simulink model "myLKS"  (R2013b)
settings: Solver=ode45  StartTime=0.0  StopTime=10.0  RelTol=1e-3
undefined symbols (not defined in the file or in its folder): A, B, GearRatio, K, L
settings Model: Creator=IVDL  LastModifiedBy=edward
settings DataIOCC: SignalLoggingSaveFormat=ModelDataLogs
settings DebuggingCC: UnderspecifiedInitializationDetection=Simplified  MultiTaskDSMMsg=warning  MultiTaskCondExecSysMsg=none  StrictBusMsg=None
settings RTWCC: IncludeERTFirstTime=on
settings GRTTargetCC: CodeReplacementLibrary=None  CPPClassGenCompliant=on

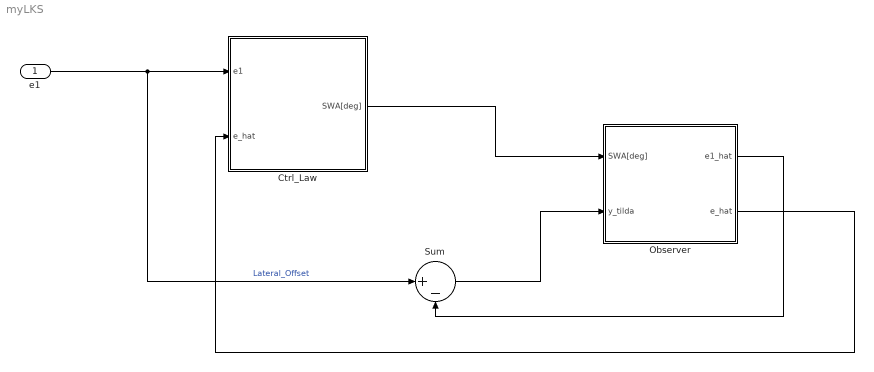
== system myLKS ==
  e1 : Inport
  Ctrl_Law : Subsystem
  Observer : Subsystem
  Sum : Sum  Inputs=|+-
  wires:
  Sum/1 -> Observer/2(y_tilda)
  e1/1 -> Sum/1, Ctrl_Law/1(e1)  "Lateral_Offset"
  Observer/2(e_hat) -> Ctrl_Law/2(e_hat)
  Ctrl_Law/1(SWA[deg]) -> Observer/1(SWA[deg])
  Observer/1(e1_hat) -> Sum/2

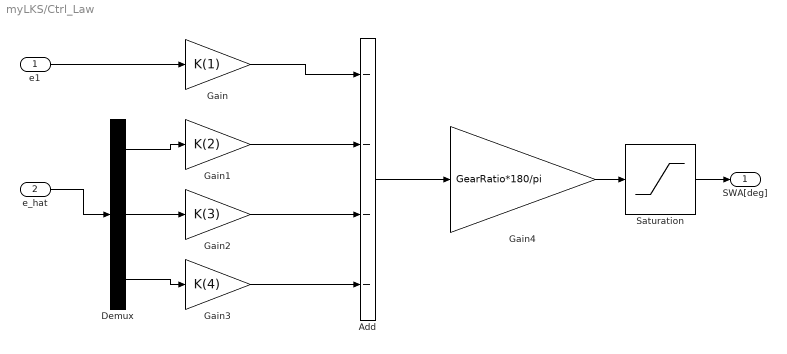
== system myLKS/Ctrl_Law ==
  e1 : Inport
  e_hat : Inport  Port=2
  Add : Sum  Inputs=----
  Demux : Demux  Outputs=3
  Gain : Gain  Gain=K(1)
  Gain1 : Gain  Gain=K(2)
  Gain2 : Gain  Gain=K(3)
  Gain3 : Gain  Gain=K(4)
  Gain4 : Gain  Gain=GearRatio*180/pi
  Saturation : Saturate
  SWA[deg] : Outport
  wires:
  Gain1/1 -> Add/2
  Gain/1 -> Add/1
  Gain4/1 -> Saturation/1
  Gain3/1 -> Add/4
  Saturation/1 -> SWA[deg]/1
  Gain2/1 -> Add/3
  Demux/2 -> Gain2/1
  Demux/3 -> Gain3/1
  e_hat/1 -> Demux/1
  Demux/1 -> Gain1/1
  e1/1 -> Gain/1
  Add/1 -> Gain4/1

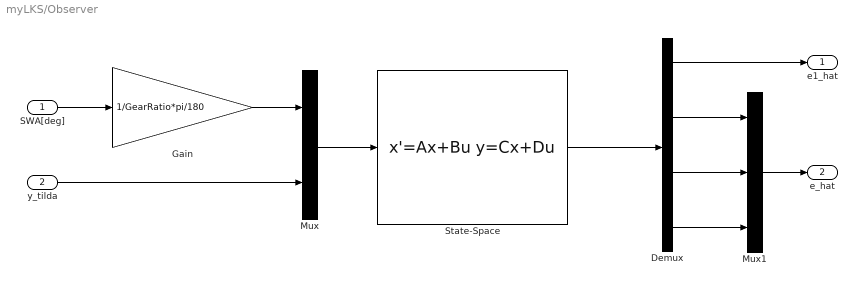
== system myLKS/Observer ==
  SWA[deg] : Inport
  y_tilda : Inport  Port=2
  Demux : Demux
  Gain : Gain  Gain=1/GearRatio*pi/180
  Mux : Mux  Inputs=2
  Mux1 : Mux  Inputs=3
  State-Space : StateSpace  A=A  B=[B L']  C=diag([1 1 1 1])  D=zeros(4,2)  X0=0  ContinuousStateAttributes={'e1','e1_dot','e2','e2_dot'}
  e1_hat : Outport
  e_hat : Outport  Port=2
  wires:
  SWA[deg]/1 -> Gain/1
  Gain/1 -> Mux/1
  y_tilda/1 -> Mux/2
  State-Space/1 -> Demux/1
  Demux/3 -> Mux1/2
  Mux1/1 -> e_hat/1
  Demux/1 -> e1_hat/1
  Mux/1 -> State-Space/1
  Demux/2 -> Mux1/1
  Demux/4 -> Mux1/3
